simulink model "TestEncoderDistancia"  (R2022b)
settings: Solver=VariableStepAuto  StartTime=0.0  StopTime=10.0  RelTol=1e-3
settings Model: Creator=Usuario  LastModifiedBy=Usuario

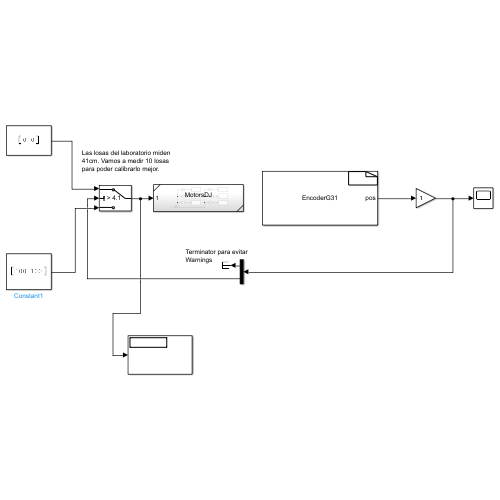
[thumbnail: Simulink's stored preview of the top-level diagram]
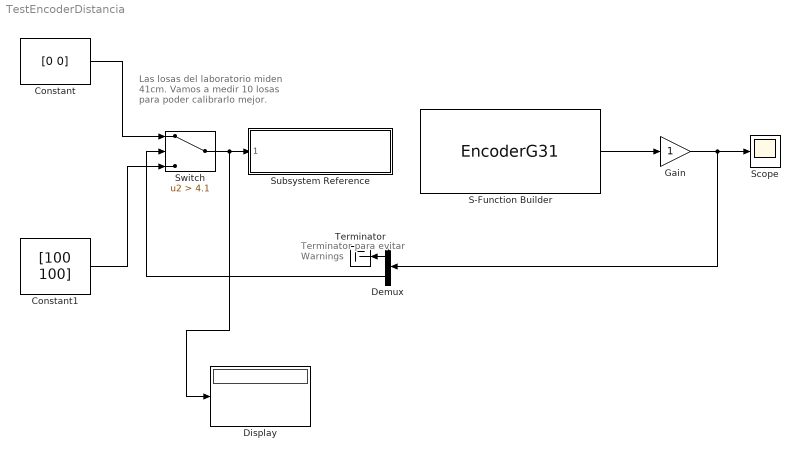
== system TestEncoderDistancia ==
  note: Terminator para evitar
      | Warnings
  note: Las losas del laboratorio miden
      | 41cm. Vamos a medir 10 losas
      | para poder calibrarlo mejor.
  Constant : Constant  Value=[0 0]  OutDataTypeStr=int16
  Constant1 : Constant  Value=[100 100]  OutDataTypeStr=int16
  Demux : Demux  Outputs=2
  Display : Display
  Gain : Gain
  S-Function Builder : S-Function  FunctionName=EncoderG31  SFunctionModules=EncoderG31_wrapper.c  SFunctionDeploymentMode=off  EnableBusSupport=off  mask(S-Function Builder){}
      mask help: Simulink:masks:SFunctionBuilder_MD
      mask init:
      | val = [[.9  0.75 0.75 1 1 .9 .9 1]',[1 1 0.75 0.75 .9 .9 1 .9]'];try , sys = get_param(gcb,'SfunBuilderFcnName');if isempty(sys), sys = get_param(gcb,'FunctionName'); end,catch, sys = get_param(gcb,'FunctionName'); end
      settings: CopyFcn=set_param(gcbh,'LinkStatus','none')  OpenFcn=sfunctionwizard(gcbh)
      mask Display:
      | plot(val(:,1),val(:,2))
      | disp(sys)
      | port_label('output',1,'pos')
  Scope : Scope
  Subsystem Reference : Subsystem  ReferencedSubsystem=MotorsDJ
  Switch : Switch  Criteria=u2 > Threshold  Threshold=4.1  SaturateOnIntegerOverflow=off  InputSameDT=off
  Terminator : Terminator
  wires:
  S-Function Builder/1 -> Gain/1
  Gain/1 -> Demux/1, Scope/1
  Switch/1 -> Display/1, Subsystem Reference/1
  Constant/1 -> Switch/1
  Constant1/1 -> Switch/3
  Demux/2 -> Switch/2
  Demux/1 -> Terminator/1
